simulink library "LIB_TF_G_111"  (Simulink 8.6)
settings: Solver=ode45  StartTime=0.0  StopTime=10.0  RelTol=1e-3
PreLoadFcn:
  | if exist('tl_preloadfcn','file'), tl_preloadfcn(gcs,402); end
PostLoadFcn:
  | if exist('tl_postloadfcn','file'), tl_postloadfcn(gcs,402); end
undefined symbols (not defined in the file or in its folder): ddv
libraries: tllib x1
CloseFcn:
  | if exist('tl_closefcn','file'), tl_closefcn(gcs); end
settings Model: TLRevision=402  Creator=cedric.sauvage  LastModifiedBy=pierre-olivier.pilot

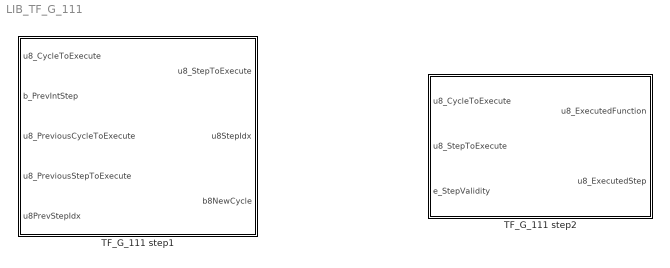
== system LIB_TF_G_111 ==
  TF_G_111 step1 : Subsystem  RequirementInfo={} %GIDa_1baf4a10_21df_4359_ba4d_6c5534378a62  TreatAsAtomicUnit=on
  TF_G_111 step2 : Subsystem  Description=The subsystemDetermineExecutedFunction block is in charge of providing the current executed function output.  RequirementInfo={} %GIDa_d7e9ae14_b57a_42d0_b34c_a685cd16cf1f  TreatAsAtomicUnit=on  RTWFcnName=SelectCycleToExecute
      settings: RTWFcnNameOpts=Use subsystem name

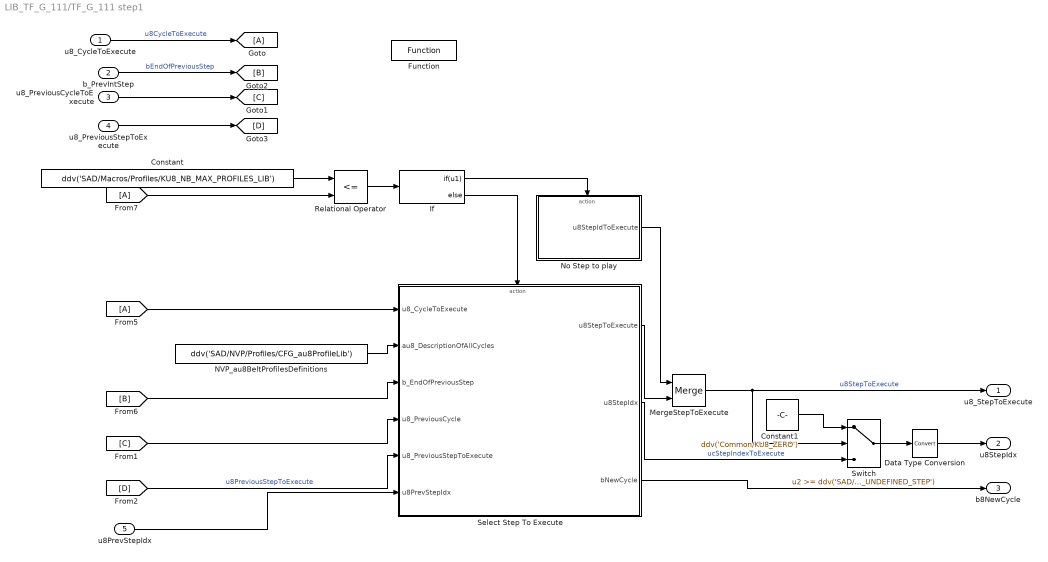
== system LIB_TF_G_111/TF_G_111 step1 ==
  u8_CycleToExecute : Inport  RequirementInfo={} %GIDa_1aab57bb_0326_4cdf_993d_e8a3d032b2dd  PortDimensions=1
  b_PrevIntStep : Inport  RequirementInfo={} %GIDa_baf42ac9_6a3f_411d_a9f1_a6624943f8b6  Port=2  PortDimensions=1
  u8_PreviousCycleToExecute : Inport  RequirementInfo={} %GIDa_c03a94d2_b76b_499f_8873_89e674a9d0bd  Port=3  PortDimensions=1
  u8_PreviousStepToExecute : Inport  RequirementInfo={} %GIDa_366c8ebc_64c9_4731_a983_8ea26311e48e  Port=4  PortDimensions=1
  u8PrevStepIdx : Inport  RequirementInfo={} %GIDa_366c8ebc_64c9_4731_a983_8ea26311e48e  Port=5  PortDimensions=1
  Constant : Constant  RequirementInfo="{}  %GIDa_620c8e9e_71b4_4391_b94d_f5bd98887c44"  Value=ddv('SAD/Macros/Profiles/KU8_NB_MAX_PROFILES_LIB')  OutDataTypeStr=uint8  mask(TL_Constant){data={'output',{'variable','SAD/Macros/Profiles/KU8_NB_MAX_PROFILES_LIB'},'date',738317.72550504631}}
      settings: CopyFcn=if exist('tl_reset_reviewflag','file')==2,tl_reset_reviewflag(gcbh);end  DeleteFcn=if exist('delete_tlblock','file')==2,delete_tlblock(gcbh);end  NameChangeFcn=if exist('rename_tlblock','file')==2,rename_tlblock(gcbh);end  OpenFcn=if exist('tl_open_blockdlg','file')==2,tl_open_blockdlg(gcbh);else,open_system(gcbh,'parameter');end
      mask Help: eval(['if exist(''tl_online_help'',''file'') == 2, tl_online_help(''Topic'',''TL_Constant''),else, web([''jar:file:///'',matlabroot,''/help/toolbox/simulink/help.jar!/slref/' lower(get_param(gcbh,'Blocktype')) '.html''], ''-helpbrowser''),end'])
      mask Display: plot([-0.05, 1.05, NaN, -0.05, 1.05],[.01, .01, NaN, .99, .99])
  Constant1 : Constant  Value=ddv('Common/KU8_ZERO')  mask(TL_Constant){data={'output',{'variable','Common/KU8_ZERO'},'date',738374.40284888889}}
      settings: CopyFcn=if exist('tl_reset_reviewflag') == 2, tl_reset_reviewflag(gcbh); end  DeleteFcn=if exist('delete_tlblock','file')==2,delete_tlblock(gcbh);end  NameChangeFcn=if exist('rename_tlblock','file')==2,rename_tlblock(gcbh);end  OpenFcn=if exist('tl_open_blockdlg','file')==2,tl_open_blockdlg(gcbh);else,open_system(gcbh,'parameter');end
      mask Help: eval(['if exist(''tl_online_help'',''file'') == 2, tl_online_help(''Topic'',''TL_Constant''),else, web([''jar:file:///'',matlabroot,''/help/toolbox/simulink/help.jar!/slref/' lower(get_param(gcbh,'Blocktype')) '.html''], ''-helpbrowser''),end'])
      mask Display: plot([-0.1, 1.05, NaN, -0.1, 1.05],[.01, .01, NaN, .99, .99]);
  Data Type Conversion : DataTypeConversion
  Function : tllib/Function  RequirementInfo={'other' '..\..\..\..\Documents and Settings\cedric.sauvage\Desktop\BFE_Design.doc' '@Simulink_requirement_item_11' 'true' 'DSG_BFE_00022' '' } %GIDa_e008078b_e0b8_4be4_b617_b81ec49ed686  data={'stepfunctionname','M_SelectStepId','stepfunctionclass','STATIC_FCN','restartfunctionname','RESTART_$S','initfunctionname','INIT_$S','termfunctionname','TERM_$S','subsystemid','b','codecomment',['[COVERS: DSG_BFE_00022]'],'date',738317.71884769679}  displayString=FUNCTION
  If : If  RequirementInfo="{}  %GIDa_294fbd4d_f0d9_4546_9a6f_38fd5f5ce9cd"  IfExpression=u1
  MergeStepToExecute : Merge  RequirementInfo={} %GIDa_00bbe0bd_4739_4f59_a29d_488204ffbd9c  InitialOutput=255  mask(TL_Merge){data={'comment',{'text',['Variable to store the Step Id that will be executed.' char(10) 'Range : [0 ; 7 ] U {255}']},'logdata',{'loggingmode',1},'output',{'name','u8StepToExecute','type','UInt8','inheritscaling',0},'autoscaling',{'mode',2},'date',738342.71431006945}}
      settings: CopyFcn=if exist('tl_reset_reviewflag','file')==2,tl_reset_reviewflag(gcbh);end  DeleteFcn=if exist('delete_tlblock','file')==2,delete_tlblock(gcbh);end  NameChangeFcn=if exist('rename_tlblock','file')==2,rename_tlblock(gcbh);end  OpenFcn=if exist('tl_open_blockdlg','file')==2,tl_open_blockdlg(gcbh);else,open_system(gcbh,'parameter');end
      mask Help: eval(['if exist(''tl_online_help'',''file'') == 2, tl_online_help(''Topic'',''TL_Merge''),else, web([''jar:file:///'',matlabroot,''/help/toolbox/simulink/help.jar!/slref/' lower(get_param(gcbh,'Blocktype')) '.html''], ''-helpbrowser''),end'])
      mask Display: plot([-0.05, 1.05, NaN, -0.05, 1.05],[.01, .01, NaN, .99, .99])
  NVP_au8BeltProfilesDefinitions : Constant  RequirementInfo={} %GIDa_2310f87e_6155_40ae_92aa_a4e85bb40bf8  Value=ddv('SAD/NVP/Profiles/CFG_au8ProfileLib')  OutDataTypeStr=uint8  SampleTime=-1  mask(TL_Constant){data={'output',{'variable','SAD/NVP/Profiles/CFG_au8ProfileLib'},'autoscaling',{'mode',2,'scalingvalid',1},'date',738317.72849901626}}
      settings: CopyFcn=if exist('tl_reset_reviewflag','file')==2,tl_reset_reviewflag(gcbh);end  DeleteFcn=if exist('delete_tlblock','file')==2,delete_tlblock(gcbh);end  NameChangeFcn=if exist('rename_tlblock','file')==2,rename_tlblock(gcbh);end  OpenFcn=if exist('tl_open_blockdlg','file')==2,tl_open_blockdlg(gcbh);else,open_system(gcbh,'parameter');end
      mask Help: eval(['if exist(''tl_online_help'',''file'') == 2, tl_online_help(''Topic'',''TL_Constant''),else, web([''jar:file:///'',matlabroot,''/help/toolbox/simulink/help.jar!/slref/' lower(get_param(gcbh,'Blocktype')) '.html''], ''-helpbrowser''),end'])
      mask Display: plot([-0.05, 1.05, NaN, -0.05, 1.05],[.01, .01, NaN, .99, .99])
  No Step to play : Subsystem  RequirementInfo={} %GIDa_d91b2e4f_18cc_4d88_b22a_15159c806b5d  TreatAsAtomicUnit=on
  Relational Operator : RelationalOperator  RequirementInfo="{}  %GIDa_efbacf4c_d6af_4eb6_a19c_9e619873ad52"  Operator=<=  OutDataTypeStr=boolean  mask(TL_RelationalOperator){data={'output',{'name','bIsValidCycle'},'date',735951.66832363431}}
      settings: DeleteFcn=if exist('delete_tlblock','file')==2,delete_tlblock(gcbh);end  NameChangeFcn=if exist('rename_tlblock','file')==2,rename_tlblock(gcbh);end  OpenFcn=if exist('tl_open_blockdlg','file')==2,tl_open_blockdlg(gcbh);else,open_system(gcbh,'parameter');end
      mask Help: eval(['if exist(''tl_online_help'',''file'') == 2, tl_online_help(''Topic'',''TL_RelationalOperator''),else, web([''jar:file:///'',matlabroot,''/help/toolbox/simulink/help.jar!/slref/' lower(get_param(gcbh,'Blocktype')) '.html''], ''-helpbrowser''),end'])
      mask Display: plot([-0.05, 1.05, NaN, -0.05, 1.05],[.01, .01, NaN, .99, .99])
  Select Step To Execute : Subsystem  RequirementInfo={} %GIDa_31ce642c_6a48_44ac_acee_58c46d748f2b  TreatAsAtomicUnit=on  RTWFcnName=SelectStepToExecute
      settings: RTWFcnNameOpts=Use subsystem name
  Switch : Switch  Threshold=ddv('SAD/Macros/Steps/KUC_UNDEFINED_STEP')  mask(TL_Switch){data={'output',{'type','UInt8'},'threshold',{'variable','SAD/Macros/Steps/KUC_UNDEFINED_STEP'},'date',738374.39737903932}}
      settings: CopyFcn=if exist('tl_reset_reviewflag') == 2, tl_reset_reviewflag(gcbh); end  DeleteFcn=if exist('delete_tlblock','file')==2,delete_tlblock(gcbh);end  NameChangeFcn=if exist('rename_tlblock','file')==2,rename_tlblock(gcbh);end  OpenFcn=if exist('tl_open_blockdlg','file')==2,tl_open_blockdlg(gcbh);else,open_system(gcbh,'parameter');end
      mask Help: eval(['if exist(''tl_online_help'',''file'') == 2, tl_online_help(''Topic'',''TL_Switch''),else, web([''jar:file:///'',matlabroot,''/help/toolbox/simulink/help.jar!/slref/' lower(get_param(gcbh,'Blocktype')) '.html''], ''-helpbrowser''),end'])
      mask Display: plot([-0.1, 1.05, NaN, -0.1, 1.05],[.01, .01, NaN, .99, .99]);
  u8_StepToExecute : Outport  RequirementInfo={} %GIDa_adc63fab_a360_486b_a74e_418a5d4fa8d3  PortDimensions=1
  u8StepIdx : Outport  RequirementInfo={} %GIDa_adc63fab_a360_486b_a74e_418a5d4fa8d3  Port=2  PortDimensions=1
  b8NewCycle : Outport  RequirementInfo={} %GIDa_adc63fab_a360_486b_a74e_418a5d4fa8d3  Port=3  PortDimensions=1
  wires:
  MergeStepToExecute/1 -> Switch/2, u8_StepToExecute/1  "u8StepToExecute"
  Select Step To Execute/1(u8StepToExecute) -> MergeStepToExecute/2
  NVP_au8BeltProfilesDefinitions/1 -> Select Step To Execute/2(au8_DescriptionOfAllCycles)
  [D] -> Select Step To Execute/5(u8_PreviousStepToExecute)  "u8PreviousStepToExecute"
  [C] -> Select Step To Execute/4(u8_PreviousCycle)
  b_PrevIntStep/1 -> [B]  "bEndOfPreviousStep"
  [A] -> Select Step To Execute/1(u8_CycleToExecute)
  [B] -> Select Step To Execute/3(b_EndOfPreviousStep)
  If/1 -> No Step to play/Action
  Constant/1 -> Relational Operator/1
  [A] -> Relational Operator/2
  Relational Operator/1 -> If/1
  If/2 -> Select Step To Execute/Action
  No Step to play/1(u8StepIdToExecute) -> MergeStepToExecute/1
  u8_PreviousCycleToExecute/1 -> [C]
  u8_PreviousStepToExecute/1 -> [D]
  u8PrevStepIdx/1 -> Select Step To Execute/6(u8PrevStepIdx)
  Switch/1 -> Data Type Conversion/1
  Select Step To Execute/2(u8StepIdx) -> Switch/3  "ucStepIndexToExecute"
  Data Type Conversion/1 -> u8StepIdx/1
  Constant1/1 -> Switch/1
  Select Step To Execute/3(bNewCycle) -> b8NewCycle/1
  u8_CycleToExecute/1 -> [A]  "u8CycleToExecute"

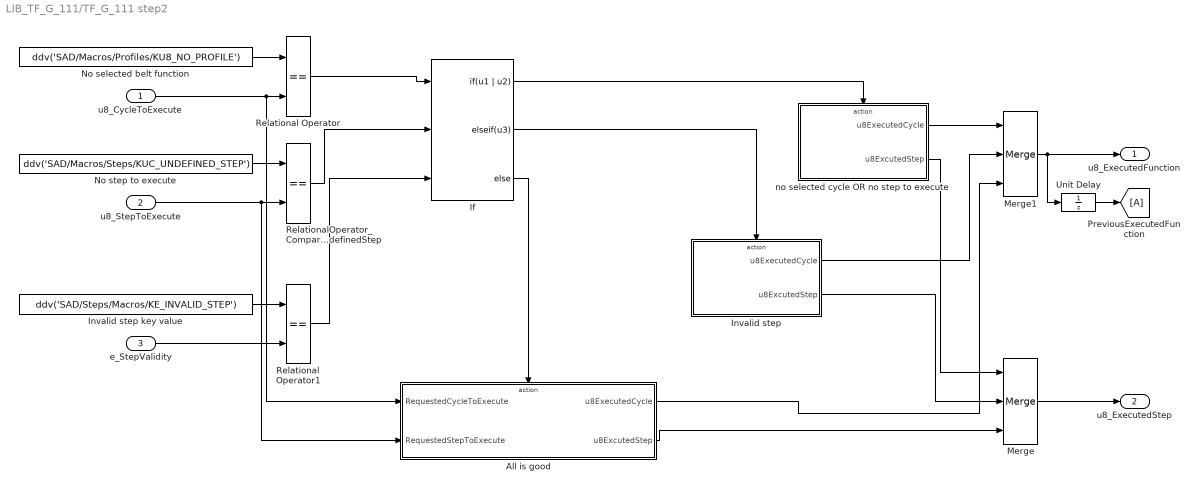
== system LIB_TF_G_111/TF_G_111 step2 ==
  u8_CycleToExecute : Inport  RequirementInfo={} %GIDa_8fea8efb_b987_405d_b9e8_745dfc9acb95
  u8_StepToExecute : Inport  RequirementInfo={} %GIDa_61957716_bf53_4143_936d_c46b278fe403  Port=2  OutDataTypeStr=uint8
  e_StepValidity : Inport  RequirementInfo={} %GIDa_5e092c6c_cd76_45bb_8082_3f7ed93fce89  Port=3
  All is good : Subsystem  TreatAsAtomicUnit=on
  If : If  NumInputs=3  IfExpression=u1 | u2  ElseIfExpressions=u3
  Invalid step : Subsystem  TreatAsAtomicUnit=on
  Invalid step key value : Constant  RequirementInfo={} %GIDa_416a43f8_dea2_4baf_bffb_a83f416ddf80  Value=ddv('SAD/Steps/Macros/KE_INVALID_STEP')  OutDataTypeStr=Inherit: Inherit via back propagation  mask(TL_Constant){data={'output',{'variable','SAD/Steps/Macros/KE_INVALID_STEP'},'date',738321.62849513884}}
      settings: CopyFcn=if exist('tl_reset_reviewflag','file')==2,tl_reset_reviewflag(gcbh);end  DeleteFcn=if exist('delete_tlblock','file')==2,delete_tlblock(gcbh);end  NameChangeFcn=if exist('rename_tlblock','file')==2,rename_tlblock(gcbh);end  OpenFcn=if exist('tl_open_blockdlg','file')==2,tl_open_blockdlg(gcbh);else,open_system(gcbh,'parameter');end
      mask Help: eval(['if exist(''tl_online_help'',''file'') == 2, tl_online_help(''Topic'',''TL_Constant''),else, web([''jar:file:///'',matlabroot,''/help/toolbox/simulink/help.jar!/slref/' lower(get_param(gcbh,'Blocktype')) '.html''], ''-helpbrowser''),end'])
      mask Display: plot([-0.05, 1.05, NaN, -0.05, 1.05],[.01, .01, NaN, .99, .99])
  Merge : Merge  Inputs=3  InitialOutput=255  mask(TL_Merge){data={'output',{'name','u8ExecutedStep'},'date',738321.62694715278}}
      settings: CopyFcn=if exist('tl_reset_reviewflag','file')==2,tl_reset_reviewflag(gcbh);end  DeleteFcn=if exist('delete_tlblock','file')==2,delete_tlblock(gcbh);end  NameChangeFcn=if exist('rename_tlblock','file')==2,rename_tlblock(gcbh);end  OpenFcn=if exist('tl_open_blockdlg','file')==2,tl_open_blockdlg(gcbh);else,open_system(gcbh,'parameter');end
      mask Help: eval(['if exist(''tl_online_help'',''file'') == 2, tl_online_help(''Topic'',''TL_Merge''),else, web([''jar:file:///'',matlabroot,''/help/toolbox/simulink/help.jar!/slref/' lower(get_param(gcbh,'Blocktype')) '.html''], ''-helpbrowser''),end'])
      mask Display: plot([-0.05, 1.05, NaN, -0.05, 1.05],[.01, .01, NaN, .99, .99])
  Merge1 : Merge  Inputs=3  InitialOutput=255  mask(TL_Merge){data={'output',{'name','u8ExecutedCycle'},'date',738321.62687034719}}
      settings: CopyFcn=if exist('tl_reset_reviewflag','file')==2,tl_reset_reviewflag(gcbh);end  DeleteFcn=if exist('delete_tlblock','file')==2,delete_tlblock(gcbh);end  NameChangeFcn=if exist('rename_tlblock','file')==2,rename_tlblock(gcbh);end  OpenFcn=if exist('tl_open_blockdlg','file')==2,tl_open_blockdlg(gcbh);else,open_system(gcbh,'parameter');end
      mask Help: eval(['if exist(''tl_online_help'',''file'') == 2, tl_online_help(''Topic'',''TL_Merge''),else, web([''jar:file:///'',matlabroot,''/help/toolbox/simulink/help.jar!/slref/' lower(get_param(gcbh,'Blocktype')) '.html''], ''-helpbrowser''),end'])
      mask Display: plot([-0.05, 1.05, NaN, -0.05, 1.05],[.01, .01, NaN, .99, .99])
  No selected belt function : Constant  RequirementInfo={} %GIDa_4bc26cfd_c29d_4ec8_a88f_554466473695  Value=ddv('SAD/Macros/Profiles/KU8_NO_PROFILE')  OutDataTypeStr=uint8  mask(TL_Constant){data={'output',{'variable','SAD/Macros/Profiles/KU8_NO_PROFILE'},'date',738321.62805532408}}
      settings: CopyFcn=if exist('tl_reset_reviewflag','file')==2,tl_reset_reviewflag(gcbh);end  DeleteFcn=if exist('delete_tlblock','file')==2,delete_tlblock(gcbh);end  NameChangeFcn=if exist('rename_tlblock','file')==2,rename_tlblock(gcbh);end  OpenFcn=if exist('tl_open_blockdlg','file')==2,tl_open_blockdlg(gcbh);else,open_system(gcbh,'parameter');end
      mask Help: eval(['if exist(''tl_online_help'',''file'') == 2, tl_online_help(''Topic'',''TL_Constant''),else, web([''jar:file:///'',matlabroot,''/help/toolbox/simulink/help.jar!/slref/' lower(get_param(gcbh,'Blocktype')) '.html''], ''-helpbrowser''),end'])
      mask Display: plot([-0.05, 1.05, NaN, -0.05, 1.05],[.01, .01, NaN, .99, .99])
  No step to execute : Constant  RequirementInfo={} %GIDa_8bc1bd8d_9fc4_41ed_9f7f_2899e2e1c57d  Value=ddv('SAD/Macros/Steps/KUC_UNDEFINED_STEP')  OutDataTypeStr=Inherit: Inherit via back propagation  mask(TL_Constant){data={'output',{'variable','SAD/Macros/Steps/KUC_UNDEFINED_STEP'},'date',738321.62822025467}}
      settings: CopyFcn=if exist('tl_reset_reviewflag','file')==2,tl_reset_reviewflag(gcbh);end  DeleteFcn=if exist('delete_tlblock','file')==2,delete_tlblock(gcbh);end  NameChangeFcn=if exist('rename_tlblock','file')==2,rename_tlblock(gcbh);end  OpenFcn=if exist('tl_open_blockdlg','file')==2,tl_open_blockdlg(gcbh);else,open_system(gcbh,'parameter');end
      mask Help: eval(['if exist(''tl_online_help'',''file'') == 2, tl_online_help(''Topic'',''TL_Constant''),else, web([''jar:file:///'',matlabroot,''/help/toolbox/simulink/help.jar!/slref/' lower(get_param(gcbh,'Blocktype')) '.html''], ''-helpbrowser''),end'])
      mask Display: plot([-0.05, 1.05, NaN, -0.05, 1.05],[.01, .01, NaN, .99, .99])
  Relational Operator : RelationalOperator  Operator===  OutDataTypeStr=boolean  mask(TL_RelationalOperator){data={'date',735951.66831112269}}
      settings: DeleteFcn=if exist('delete_tlblock','file')==2,delete_tlblock(gcbh);end  NameChangeFcn=if exist('rename_tlblock','file')==2,rename_tlblock(gcbh);end  OpenFcn=if exist('tl_open_blockdlg','file')==2,tl_open_blockdlg(gcbh);else,open_system(gcbh,'parameter');end
      mask Help: eval(['if exist(''tl_online_help'',''file'') == 2, tl_online_help(''Topic'',''TL_RelationalOperator''),else, web([''jar:file:///'',matlabroot,''/help/toolbox/simulink/help.jar!/slref/' lower(get_param(gcbh,'Blocktype')) '.html''], ''-helpbrowser''),end'])
      mask Display: plot([-0.05, 1.05, NaN, -0.05, 1.05],[.01, .01, NaN, .99, .99])
  Relational Operator1 : RelationalOperator  Operator===  OutDataTypeStr=boolean  mask(TL_RelationalOperator){data={'date',735951.66831087961}}
      settings: DeleteFcn=if exist('delete_tlblock','file')==2,delete_tlblock(gcbh);end  NameChangeFcn=if exist('rename_tlblock','file')==2,rename_tlblock(gcbh);end  OpenFcn=if exist('tl_open_blockdlg','file')==2,tl_open_blockdlg(gcbh);else,open_system(gcbh,'parameter');end
      mask Help: eval(['if exist(''tl_online_help'',''file'') == 2, tl_online_help(''Topic'',''TL_RelationalOperator''),else, web([''jar:file:///'',matlabroot,''/help/toolbox/simulink/help.jar!/slref/' lower(get_param(gcbh,'Blocktype')) '.html''], ''-helpbrowser''),end'])
      mask Display: plot([-0.05, 1.05, NaN, -0.05, 1.05],[.01, .01, NaN, .99, .99])
  RelationalOperator_CompareToUndefinedStep : RelationalOperator  RequirementInfo={} %GIDa_4071e895_5093_4781_8864_58a78a6d4067  Operator===  OutDataTypeStr=boolean  mask(TL_RelationalOperator){data={'date',735951.66831063654}}
      settings: DeleteFcn=if exist('delete_tlblock','file')==2,delete_tlblock(gcbh);end  NameChangeFcn=if exist('rename_tlblock','file')==2,rename_tlblock(gcbh);end  OpenFcn=if exist('tl_open_blockdlg','file')==2,tl_open_blockdlg(gcbh);else,open_system(gcbh,'parameter');end
      mask Help: eval(['if exist(''tl_online_help'',''file'') == 2, tl_online_help(''Topic'',''TL_RelationalOperator''),else, web([''jar:file:///'',matlabroot,''/help/toolbox/simulink/help.jar!/slref/' lower(get_param(gcbh,'Blocktype')) '.html''], ''-helpbrowser''),end'])
      mask Display: plot([-0.05, 1.05, NaN, -0.05, 1.05],[.01, .01, NaN, .99, .99])
  Unit Delay : UnitDelay  InitialCondition=255  SampleTime=-1  mask(TL_UnitDelay){data={'output',{'type','UInt8'},'state',{'name','u8PreviousExecutedFunction','type','UInt8'},'date',735951.66831032408}}
      settings: CopyFcn=if exist('tl_reset_reviewflag','file')==2,tl_reset_reviewflag(gcbh);end  DeleteFcn=if exist('delete_tlblock','file')==2,delete_tlblock(gcbh);end  NameChangeFcn=if exist('rename_tlblock','file')==2,rename_tlblock(gcbh);end  OpenFcn=if exist('tl_open_blockdlg','file')==2,tl_open_blockdlg(gcbh);else,open_system(gcbh,'parameter');end
      mask Help: eval(['if exist(''tl_online_help'',''file'') == 2, tl_online_help(''Topic'',''TL_UnitDelay''),else, web([''jar:file:///'',matlabroot,''/help/toolbox/simulink/help.jar!/slref/' lower(get_param(gcbh,'Blocktype')) '.html''], ''-helpbrowser''),end'])
      mask Display: plot([-0.05, 1.05, NaN, -0.05, 1.05],[.01, .01, NaN, .99, .99])
  no selected cycle OR no step to execute : Subsystem  TreatAsAtomicUnit=on
  u8_ExecutedFunction : Outport  RequirementInfo={} %GIDa_8713064f_f4a9_42db_8bb1_59bc8ff89bda
  u8_ExecutedStep : Outport  RequirementInfo={} %GIDa_27e8687a_de30_4ff7_b10f_aecac094b4c1  Port=2
  wires:
  No selected belt function/1 -> Relational Operator/1
  u8_CycleToExecute/1 -> Relational Operator/2, All is good/1(RequestedCycleToExecute)
  No step to execute/1 -> RelationalOperator_CompareToUndefinedStep/1
  u8_StepToExecute/1 -> RelationalOperator_CompareToUndefinedStep/2, All is good/2(RequestedStepToExecute)
  If/1 -> no selected cycle OR no step to execute/Action
  Relational Operator/1 -> If/1
  RelationalOperator_CompareToUndefinedStep/1 -> If/2
  e_StepValidity/1 -> Relational Operator1/2
  Relational Operator1/1 -> If/3
  Invalid step key value/1 -> Relational Operator1/1
  If/2 -> Invalid step/Action
  If/3 -> All is good/Action
  Merge1/1 -> u8_ExecutedFunction/1, Unit Delay/1
  Merge/1 -> u8_ExecutedStep/1
  no selected cycle OR no step to execute/1(u8ExecutedCycle) -> Merge1/1
  Invalid step/1(u8ExecutedCycle) -> Merge1/2
  All is good/1(u8ExecutedCycle) -> Merge1/3
  All is good/2(u8ExcutedStep) -> Merge/3
  Invalid step/2(u8ExcutedStep) -> Merge/2
  no selected cycle OR no step to execute/2(u8ExcutedStep) -> Merge/1
  Unit Delay/1 -> [A]

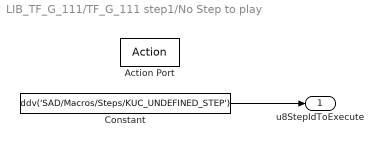
== system LIB_TF_G_111/TF_G_111 step1/No Step to play ==
  Action Port : ActionPort  RequirementInfo="{}  %GIDa_9b0f36a1_581d_4938_a95d_cea0f15c05a5"
  Constant : Constant  RequirementInfo="{}  %GIDa_afeedc86_4d10_4281_9703_4ed2f747546e"  Value=ddv('SAD/Macros/Steps/KUC_UNDEFINED_STEP')  OutDataTypeStr=uint8  mask(TL_Constant){data={'output',{'variable','SAD/Macros/Steps/KUC_UNDEFINED_STEP'},'date',738321.62035557872}}
      settings: CopyFcn=if exist('tl_reset_reviewflag','file')==2,tl_reset_reviewflag(gcbh);end  DeleteFcn=if exist('delete_tlblock','file')==2,delete_tlblock(gcbh);end  NameChangeFcn=if exist('rename_tlblock','file')==2,rename_tlblock(gcbh);end  OpenFcn=if exist('tl_open_blockdlg','file')==2,tl_open_blockdlg(gcbh);else,open_system(gcbh,'parameter');end
      mask Help: eval(['if exist(''tl_online_help'',''file'') == 2, tl_online_help(''Topic'',''TL_Constant''),else, web([''jar:file:///'',matlabroot,''/help/toolbox/simulink/help.jar!/slref/' lower(get_param(gcbh,'Blocktype')) '.html''], ''-helpbrowser''),end'])
      mask Display: plot([-0.05, 1.05, NaN, -0.05, 1.05],[.01, .01, NaN, .99, .99])
  u8StepIdToExecute : Outport  RequirementInfo={} %GIDa_e4a2b18c_09f1_4793_aba0_5f1c3953a216  InitialOutput=255
  wires:
  Constant/1 -> u8StepIdToExecute/1

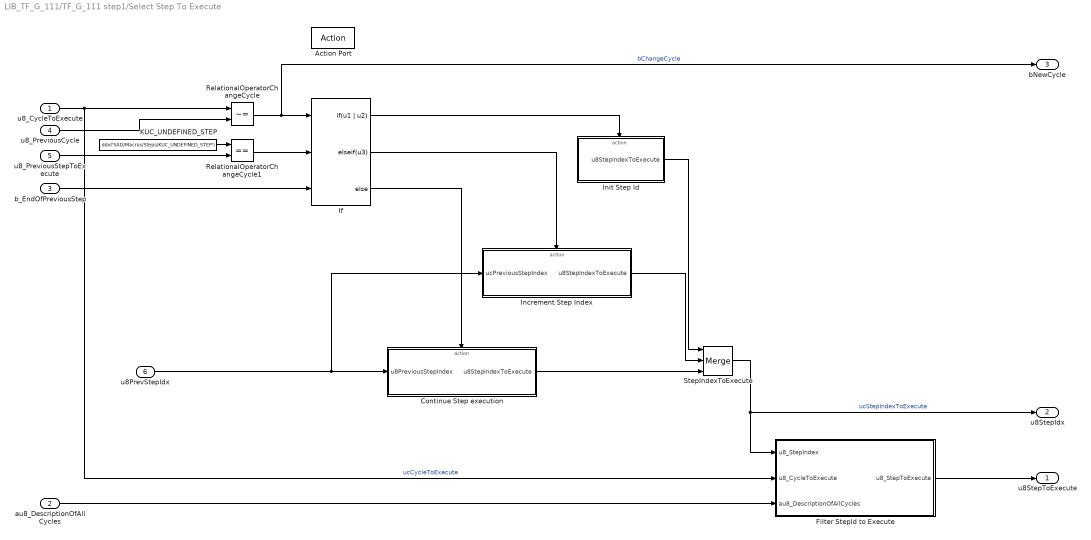
== system LIB_TF_G_111/TF_G_111 step1/Select Step To Execute ==
  u8_CycleToExecute : Inport  RequirementInfo={} %GIDa_8d4e5bab_b80e_4e01_81ce_b6e790b131fb
  au8_DescriptionOfAllCycles : Inport  RequirementInfo={} %GIDa_c06da474_c08f_46d9_92bb_9088ec013155  Port=2  OutDataTypeStr=uint8
  b_EndOfPreviousStep : Inport  RequirementInfo={} %GIDa_2c1722e4_980a_48a1_8990_301358730051  Port=3
  u8_PreviousCycle : Inport  RequirementInfo={} %GIDa_7ceb08ad_35fc_4b74_8f3b_a28497a2e219  Port=4
  u8_PreviousStepToExecute : Inport  RequirementInfo={} %GIDa_3793ab51_f047_4f43_8cee_9c5d044f6ee6  Port=5
  u8PrevStepIdx : Inport  RequirementInfo={} %GIDa_c06da474_c08f_46d9_92bb_9088ec013155  Port=6
  Action Port : ActionPort  RequirementInfo="{}  %GIDa_ec02541f_ac93_4bf3_836c_122371ae3eb9"
  Continue Step execution : Subsystem  RequirementInfo={} %GIDa_567d5d98_645d_41b3_b901_4f423276d610  TreatAsAtomicUnit=on
      settings: RTWFcnNameOpts=Use subsystem name
  Filter StepId to Execute : Subsystem  RequirementInfo="{}  %GIDa_085e2bbf_61cb_45fc_84b4_da4c9f215240"  TreatAsAtomicUnit=on
  If : If  RequirementInfo="{}  %GIDa_fe303313_68dd_49c9_a488_ab8c67144df8"  NumInputs=3  IfExpression=u1 | u2  ElseIfExpressions=u3
  Increment Step Index : Subsystem  RequirementInfo={} %GIDa_2230e77a_bf9c_4d74_97b3_452ba0c63b0a  TreatAsAtomicUnit=on
      settings: RTWFcnNameOpts=Use subsystem name
  Init Step Id : Subsystem  RequirementInfo={} %GIDa_4cdf07f5_0d4f_4f30_b6c8_d016748c9874  TreatAsAtomicUnit=on
      settings: RTWFcnNameOpts=Use subsystem name
  KUC_UNDEFINED_STEP : Constant  RequirementInfo={} %GIDa_15357e27_e5c7_4390_bd4f_b839d31ef5c6  Value=ddv('SAD/Macros/Steps/KUC_UNDEFINED_STEP')  OutDataTypeStr=uint8  mask(TL_Constant){data={'output',{'variable','SAD/Macros/Steps/KUC_UNDEFINED_STEP'},'date',738321.62077575235}}
      settings: CopyFcn=if exist('tl_reset_reviewflag','file')==2,tl_reset_reviewflag(gcbh);end  DeleteFcn=if exist('delete_tlblock','file')==2,delete_tlblock(gcbh);end  NameChangeFcn=if exist('rename_tlblock','file')==2,rename_tlblock(gcbh);end  OpenFcn=if exist('tl_open_blockdlg','file')==2,tl_open_blockdlg(gcbh);else,open_system(gcbh,'parameter');end
      mask Help: eval(['if exist(''tl_online_help'',''file'') == 2, tl_online_help(''Topic'',''TL_Constant''),else, web([''jar:file:///'',matlabroot,''/help/toolbox/simulink/help.jar!/slref/' lower(get_param(gcbh,'Blocktype')) '.html''], ''-helpbrowser''),end'])
      mask Display: plot([-0.05, 1.05, NaN, -0.05, 1.05],[.01, .01, NaN, .99, .99])
  RelationalOperatorChangeCycle : RelationalOperator  RequirementInfo={} %GIDa_0c82807a_81d1_42ec_adac_a2f1c288664a  Operator=~=  OutDataTypeStr=boolean  ZeroCross=off  mask(TL_RelationalOperator){data={'output',{'name','bHasCycleChanged'},'date',735951.66831762728}}
      settings: DeleteFcn=if exist('delete_tlblock','file')==2,delete_tlblock(gcbh);end  NameChangeFcn=if exist('rename_tlblock','file')==2,rename_tlblock(gcbh);end  OpenFcn=if exist('tl_open_blockdlg','file')==2,tl_open_blockdlg(gcbh);else,open_system(gcbh,'parameter');end
      mask Help: eval(['if exist(''tl_online_help'',''file'') == 2, tl_online_help(''Topic'',''TL_RelationalOperator''),else, web([''jar:file:///'',matlabroot,''/help/toolbox/simulink/help.jar!/slref/' lower(get_param(gcbh,'Blocktype')) '.html''], ''-helpbrowser''),end'])
      mask Display: plot([-0.05, 1.05, NaN, -0.05, 1.05],[.01, .01, NaN, .99, .99])
  RelationalOperatorChangeCycle1 : RelationalOperator  RequirementInfo={} %GIDa_c96d9746_f8c6_4abd_a58c_f9e69e7c3389  Operator===  OutDataTypeStr=boolean  ZeroCross=off  mask(TL_RelationalOperator){data={'date',735951.66831736115}}
      settings: DeleteFcn=if exist('delete_tlblock','file')==2,delete_tlblock(gcbh);end  NameChangeFcn=if exist('rename_tlblock','file')==2,rename_tlblock(gcbh);end  OpenFcn=if exist('tl_open_blockdlg','file')==2,tl_open_blockdlg(gcbh);else,open_system(gcbh,'parameter');end
      mask Help: eval(['if exist(''tl_online_help'',''file'') == 2, tl_online_help(''Topic'',''TL_RelationalOperator''),else, web([''jar:file:///'',matlabroot,''/help/toolbox/simulink/help.jar!/slref/' lower(get_param(gcbh,'Blocktype')) '.html''], ''-helpbrowser''),end'])
      mask Display: plot([-0.05, 1.05, NaN, -0.05, 1.05],[.01, .01, NaN, .99, .99])
  StepIndexToExecute : Merge  RequirementInfo={} %GIDa_1b7985cc_8fad_4670_b396_0d4aca6974d8  Inputs=3  InitialOutput=255  mask(TL_Merge){data={'output',{'name','u8UnfilteredStepId'},'date',735951.66831707174}}
      settings: CopyFcn=if exist('tl_reset_reviewflag','file')==2,tl_reset_reviewflag(gcbh);end  DeleteFcn=if exist('delete_tlblock','file')==2,delete_tlblock(gcbh);end  NameChangeFcn=if exist('rename_tlblock','file')==2,rename_tlblock(gcbh);end  OpenFcn=if exist('tl_open_blockdlg','file')==2,tl_open_blockdlg(gcbh);else,open_system(gcbh,'parameter');end
      mask Help: eval(['if exist(''tl_online_help'',''file'') == 2, tl_online_help(''Topic'',''TL_Merge''),else, web([''jar:file:///'',matlabroot,''/help/toolbox/simulink/help.jar!/slref/' lower(get_param(gcbh,'Blocktype')) '.html''], ''-helpbrowser''),end'])
      mask Display: plot([-0.05, 1.05, NaN, -0.05, 1.05],[.01, .01, NaN, .99, .99])
  u8StepToExecute : Outport  RequirementInfo={} %GIDa_433c26c1_7119_4ede_b400_eae74db2e302  InitialOutput=255
  u8StepIdx : Outport  RequirementInfo={} %GIDa_433c26c1_7119_4ede_b400_eae74db2e302  Port=2  InitialOutput=255
  bNewCycle : Outport  RequirementInfo={} %GIDa_433c26c1_7119_4ede_b400_eae74db2e302  Port=3  InitialOutput=0
  wires:
  b_EndOfPreviousStep/1 -> If/3
  StepIndexToExecute/1 -> Filter StepId to Execute/1(u8_StepIndex), u8StepIdx/1  "ucStepIndexToExecute"
  Increment Step Index/1(u8StepIndexToExecute) -> StepIndexToExecute/2
  u8_CycleToExecute/1 -> RelationalOperatorChangeCycle/1, Filter StepId to Execute/2(u8_CycleToExecute)  "ucCycleToExecute"
  Init Step Id/1(u8StepIndexToExecute) -> StepIndexToExecute/1
  u8_PreviousCycle/1 -> RelationalOperatorChangeCycle/2
  u8_PreviousStepToExecute/1 -> RelationalOperatorChangeCycle1/2
  RelationalOperatorChangeCycle/1 -> bNewCycle/1, If/1  "bChangeCycle"
  If/1 -> Init Step Id/Action
  If/2 -> Increment Step Index/Action
  If/3 -> Continue Step execution/Action
  KUC_UNDEFINED_STEP/1 -> RelationalOperatorChangeCycle1/1
  RelationalOperatorChangeCycle1/1 -> If/2
  Continue Step execution/1(u8StepIndexToExecute) -> StepIndexToExecute/3
  au8_DescriptionOfAllCycles/1 -> Filter StepId to Execute/3(au8_DescriptionOfAllCycles)
  u8PrevStepIdx/1 -> Increment Step Index/1(ucPreviousStepIndex), Continue Step execution/1(u8PreviousStepIndex)
  Filter StepId to Execute/1(u8_StepToExecute) -> u8StepToExecute/1

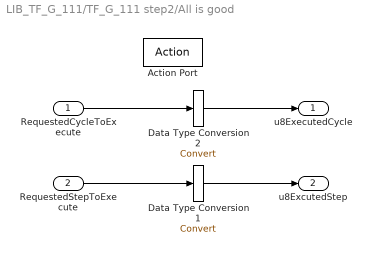
== system LIB_TF_G_111/TF_G_111 step2/All is good ==
  RequestedCycleToExecute : Inport  RequirementInfo={} %GIDa_c6656af6_5dc6_4240_9dfe_354d08ac5268
  RequestedStepToExecute : Inport  RequirementInfo={} %GIDa_947e64c1_bf3b_4bd6_a910_13dfd1c197d6  Port=2  OutDataTypeStr=uint8
  Action Port : ActionPort  ActionType=else
  Data Type Conversion1 : DataTypeConversion
  Data Type Conversion2 : DataTypeConversion
  u8ExecutedCycle : Outport
  u8ExcutedStep : Outport  Port=2
  wires:
  RequestedCycleToExecute/1 -> Data Type Conversion2/1
  RequestedStepToExecute/1 -> Data Type Conversion1/1
  Data Type Conversion2/1 -> u8ExecutedCycle/1
  Data Type Conversion1/1 -> u8ExcutedStep/1

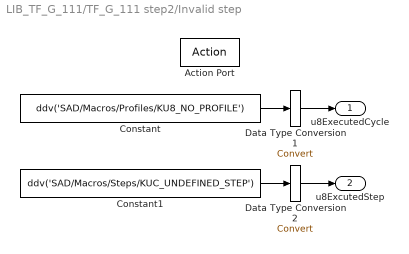
== system LIB_TF_G_111/TF_G_111 step2/Invalid step ==
  Action Port : ActionPort  ActionType=elseif
  Constant : Constant  Value=ddv('SAD/Macros/Profiles/KU8_NO_PROFILE')  mask(TL_Constant){data={'output',{'variable','SAD/Macros/Profiles/KU8_NO_PROFILE'},'date',738321.62969498837}}
      settings: CopyFcn=if exist('tl_reset_reviewflag','file')==2,tl_reset_reviewflag(gcbh);end  DeleteFcn=if exist('delete_tlblock','file')==2,delete_tlblock(gcbh);end  NameChangeFcn=if exist('rename_tlblock','file')==2,rename_tlblock(gcbh);end  OpenFcn=if exist('tl_open_blockdlg','file')==2,tl_open_blockdlg(gcbh);else,open_system(gcbh,'parameter');end
      mask Help: eval(['if exist(''tl_online_help'',''file'') == 2, tl_online_help(''Topic'',''TL_Constant''),else, web([''jar:file:///'',matlabroot,''/help/toolbox/simulink/help.jar!/slref/' lower(get_param(gcbh,'Blocktype')) '.html''], ''-helpbrowser''),end'])
      mask Display: plot([-0.05, 1.05, NaN, -0.05, 1.05],[.01, .01, NaN, .99, .99])
  Constant1 : Constant  Value=ddv('SAD/Macros/Steps/KUC_UNDEFINED_STEP')  mask(TL_Constant){data={'output',{'variable','SAD/Macros/Steps/KUC_UNDEFINED_STEP'},'date',738321.62986325228}}
      settings: CopyFcn=if exist('tl_reset_reviewflag','file')==2,tl_reset_reviewflag(gcbh);end  DeleteFcn=if exist('delete_tlblock','file')==2,delete_tlblock(gcbh);end  NameChangeFcn=if exist('rename_tlblock','file')==2,rename_tlblock(gcbh);end  OpenFcn=if exist('tl_open_blockdlg','file')==2,tl_open_blockdlg(gcbh);else,open_system(gcbh,'parameter');end
      mask Help: eval(['if exist(''tl_online_help'',''file'') == 2, tl_online_help(''Topic'',''TL_Constant''),else, web([''jar:file:///'',matlabroot,''/help/toolbox/simulink/help.jar!/slref/' lower(get_param(gcbh,'Blocktype')) '.html''], ''-helpbrowser''),end'])
      mask Display: plot([-0.05, 1.05, NaN, -0.05, 1.05],[.01, .01, NaN, .99, .99])
  Data Type Conversion1 : DataTypeConversion
  Data Type Conversion2 : DataTypeConversion
  u8ExecutedCycle : Outport
  u8ExcutedStep : Outport  Port=2
  wires:
  Constant1/1 -> Data Type Conversion2/1
  Constant/1 -> Data Type Conversion1/1
  Data Type Conversion1/1 -> u8ExecutedCycle/1
  Data Type Conversion2/1 -> u8ExcutedStep/1

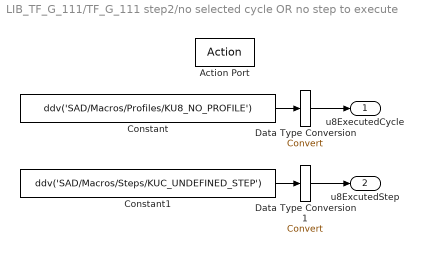
== system LIB_TF_G_111/TF_G_111 step2/no selected cycle OR no step to execute ==
  Action Port : ActionPort
  Constant : Constant  Value=ddv('SAD/Macros/Profiles/KU8_NO_PROFILE')  mask(TL_Constant){data={'output',{'variable','SAD/Macros/Profiles/KU8_NO_PROFILE'},'date',738321.62906249997}}
      settings: CopyFcn=if exist('tl_reset_reviewflag','file')==2,tl_reset_reviewflag(gcbh);end  DeleteFcn=if exist('delete_tlblock','file')==2,delete_tlblock(gcbh);end  NameChangeFcn=if exist('rename_tlblock','file')==2,rename_tlblock(gcbh);end  OpenFcn=if exist('tl_open_blockdlg','file')==2,tl_open_blockdlg(gcbh);else,open_system(gcbh,'parameter');end
      mask Help: eval(['if exist(''tl_online_help'',''file'') == 2, tl_online_help(''Topic'',''TL_Constant''),else, web([''jar:file:///'',matlabroot,''/help/toolbox/simulink/help.jar!/slref/' lower(get_param(gcbh,'Blocktype')) '.html''], ''-helpbrowser''),end'])
      mask Display: plot([-0.05, 1.05, NaN, -0.05, 1.05],[.01, .01, NaN, .99, .99])
  Constant1 : Constant  Value=ddv('SAD/Macros/Steps/KUC_UNDEFINED_STEP')  mask(TL_Constant){data={'output',{'variable','SAD/Macros/Steps/KUC_UNDEFINED_STEP'},'date',738321.62919261574}}
      settings: CopyFcn=if exist('tl_reset_reviewflag','file')==2,tl_reset_reviewflag(gcbh);end  DeleteFcn=if exist('delete_tlblock','file')==2,delete_tlblock(gcbh);end  NameChangeFcn=if exist('rename_tlblock','file')==2,rename_tlblock(gcbh);end  OpenFcn=if exist('tl_open_blockdlg','file')==2,tl_open_blockdlg(gcbh);else,open_system(gcbh,'parameter');end
      mask Help: eval(['if exist(''tl_online_help'',''file'') == 2, tl_online_help(''Topic'',''TL_Constant''),else, web([''jar:file:///'',matlabroot,''/help/toolbox/simulink/help.jar!/slref/' lower(get_param(gcbh,'Blocktype')) '.html''], ''-helpbrowser''),end'])
      mask Display: plot([-0.05, 1.05, NaN, -0.05, 1.05],[.01, .01, NaN, .99, .99])
  Data Type Conversion : DataTypeConversion
  Data Type Conversion1 : DataTypeConversion
  u8ExecutedCycle : Outport
  u8ExcutedStep : Outport  Port=2
  wires:
  Constant/1 -> Data Type Conversion/1
  Constant1/1 -> Data Type Conversion1/1
  Data Type Conversion/1 -> u8ExecutedCycle/1
  Data Type Conversion1/1 -> u8ExcutedStep/1

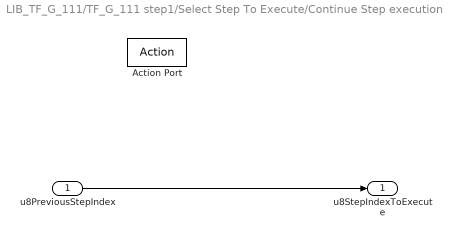
== system LIB_TF_G_111/TF_G_111 step1/Select Step To Execute/Continue Step execution ==
  u8PreviousStepIndex : Inport  RequirementInfo={} %GIDa_fcab27a8_d90a_476c_90c0_241a1e619ec6
  Action Port : ActionPort  RequirementInfo="{}  %GIDa_2c9213f9_d16e_4c91_b642_aee43e9521f1"
  u8StepIndexToExecute : Outport  RequirementInfo={} %GIDa_e09eef44_9847_4a18_ad42_ef98529f821c  InitialOutput=0
  wires:
  u8PreviousStepIndex/1 -> u8StepIndexToExecute/1

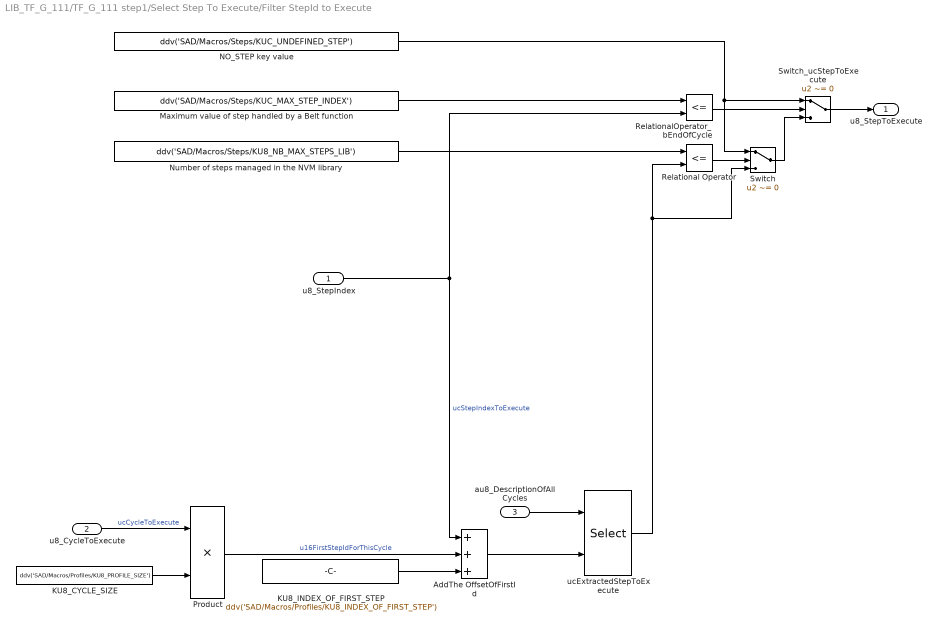
== system LIB_TF_G_111/TF_G_111 step1/Select Step To Execute/Filter StepId to Execute ==
  u8_StepIndex : Inport  RequirementInfo={} %GIDa_7b053a8d_c52f_4f18_a513_21b4e1d02a17  OutDataTypeStr=uint8
  u8_CycleToExecute : Inport  RequirementInfo={} %GIDa_17b8980e_413a_49cb_bbdf_19e5995df7c7  Port=2
  au8_DescriptionOfAllCycles : Inport  RequirementInfo={} %GIDa_914676ae_5bff_4223_821e_99fcbbab0d97  Port=3  OutDataTypeStr=uint8
  AddThe OffsetOfFirstId : Sum  RequirementInfo={} %GIDa_103df495_b24f_4135_8450_3ac2a6ce6256  Inputs=+++  SaturateOnIntegerOverflow=on  OutDataTypeStr=Inherit: Same as first input  mask(TL_Sum){data={'output',{'name','u16StepBytePosition','class','MERGEABLE_GLOBAL','type','UInt16'},'date',738322.64736040507}}
      settings: CopyFcn=if exist('tl_reset_reviewflag','file')==2,tl_reset_reviewflag(gcbh);end  DeleteFcn=if exist('delete_tlblock','file')==2,delete_tlblock(gcbh);end  NameChangeFcn=if exist('rename_tlblock','file')==2,rename_tlblock(gcbh);end  OpenFcn=if exist('tl_open_blockdlg','file')==2,tl_open_blockdlg(gcbh);else,open_system(gcbh,'parameter');end
      mask Help: eval(['if exist(''tl_online_help'',''file'') == 2, tl_online_help(''Topic'',''TL_Sum''),else, web([''jar:file:///'',matlabroot,''/help/toolbox/simulink/help.jar!/slref/' lower(get_param(gcbh,'Blocktype')) '.html''], ''-helpbrowser''),end'])
      mask Display: plot([-0.05, 1.05, NaN, -0.05, 1.05],[.01, .01, NaN, .99, .99])
  KU8_CYCLE_SIZE : Constant  RequirementInfo={} %GIDa_08c4f1ca_bb09_405a_a089_057d29aeb7e1  Value=ddv('SAD/Macros/Profiles/KU8_PROFILE_SIZE')  OutDataTypeStr=Inherit: Inherit via back propagation  mask(TL_Constant){data={'output',{'variable','SAD/Macros/Profiles/KU8_PROFILE_SIZE'},'date',738321.62223840272}}
      settings: CopyFcn=if exist('tl_reset_reviewflag','file')==2,tl_reset_reviewflag(gcbh);end  DeleteFcn=if exist('delete_tlblock','file')==2,delete_tlblock(gcbh);end  NameChangeFcn=if exist('rename_tlblock','file')==2,rename_tlblock(gcbh);end  OpenFcn=if exist('tl_open_blockdlg','file')==2,tl_open_blockdlg(gcbh);else,open_system(gcbh,'parameter');end
      mask Help: eval(['if exist(''tl_online_help'',''file'') == 2, tl_online_help(''Topic'',''TL_Constant''),else, web([''jar:file:///'',matlabroot,''/help/toolbox/simulink/help.jar!/slref/' lower(get_param(gcbh,'Blocktype')) '.html''], ''-helpbrowser''),end'])
      mask Display: plot([-0.05, 1.05, NaN, -0.05, 1.05],[.01, .01, NaN, .99, .99])
  KU8_INDEX_OF_FIRST_STEP : Constant  RequirementInfo={} %GIDa_9066d25c_f8b2_4239_a924_97fad3ec8118  Value=ddv('SAD/Macros/Profiles/KU8_INDEX_OF_FIRST_STEP')  OutDataTypeStr=Inherit: Inherit via back propagation  mask(TL_Constant){data={'output',{'variable','SAD/Macros/Profiles/KU8_INDEX_OF_FIRST_STEP'},'date',738321.62240005785}}
      settings: CopyFcn=if exist('tl_reset_reviewflag','file')==2,tl_reset_reviewflag(gcbh);end  DeleteFcn=if exist('delete_tlblock','file')==2,delete_tlblock(gcbh);end  NameChangeFcn=if exist('rename_tlblock','file')==2,rename_tlblock(gcbh);end  OpenFcn=if exist('tl_open_blockdlg','file')==2,tl_open_blockdlg(gcbh);else,open_system(gcbh,'parameter');end
      mask Help: eval(['if exist(''tl_online_help'',''file'') == 2, tl_online_help(''Topic'',''TL_Constant''),else, web([''jar:file:///'',matlabroot,''/help/toolbox/simulink/help.jar!/slref/' lower(get_param(gcbh,'Blocktype')) '.html''], ''-helpbrowser''),end'])
      mask Display: plot([-0.05, 1.05, NaN, -0.05, 1.05],[.01, .01, NaN, .99, .99])
  Maximum value of step handled by a Belt function : Constant  RequirementInfo={} %GIDa_85e693c4_096a_4e13_a3eb_10d8a1b4db74  Value=ddv('SAD/Macros/Steps/KUC_MAX_STEP_INDEX')  OutDataTypeStr=Inherit: Inherit via back propagation  mask(TL_Constant){data={'output',{'variable','SAD/Macros/Steps/KUC_MAX_STEP_INDEX'},'date',738321.62344370375}}
      settings: CopyFcn=if exist('tl_reset_reviewflag','file')==2,tl_reset_reviewflag(gcbh);end  DeleteFcn=if exist('delete_tlblock','file')==2,delete_tlblock(gcbh);end  NameChangeFcn=if exist('rename_tlblock','file')==2,rename_tlblock(gcbh);end  OpenFcn=if exist('tl_open_blockdlg','file')==2,tl_open_blockdlg(gcbh);else,open_system(gcbh,'parameter');end
      mask Help: eval(['if exist(''tl_online_help'',''file'') == 2, tl_online_help(''Topic'',''TL_Constant''),else, web([''jar:file:///'',matlabroot,''/help/toolbox/simulink/help.jar!/slref/' lower(get_param(gcbh,'Blocktype')) '.html''], ''-helpbrowser''),end'])
      mask Display: plot([-0.05, 1.05, NaN, -0.05, 1.05],[.01, .01, NaN, .99, .99])
  NO_STEP key value : Constant  RequirementInfo={} %GIDa_cb4e9d1a_f250_4569_85fb_c4d5025ec8c8  Value=ddv('SAD/Macros/Steps/KUC_UNDEFINED_STEP')  OutDataTypeStr=uint8  mask(TL_Constant){data={'output',{'variable','SAD/Macros/Steps/KUC_UNDEFINED_STEP'},'date',738321.62358545139}}
      settings: CopyFcn=if exist('tl_reset_reviewflag','file')==2,tl_reset_reviewflag(gcbh);end  DeleteFcn=if exist('delete_tlblock','file')==2,delete_tlblock(gcbh);end  NameChangeFcn=if exist('rename_tlblock','file')==2,rename_tlblock(gcbh);end  OpenFcn=if exist('tl_open_blockdlg','file')==2,tl_open_blockdlg(gcbh);else,open_system(gcbh,'parameter');end
      mask Help: eval(['if exist(''tl_online_help'',''file'') == 2, tl_online_help(''Topic'',''TL_Constant''),else, web([''jar:file:///'',matlabroot,''/help/toolbox/simulink/help.jar!/slref/' lower(get_param(gcbh,'Blocktype')) '.html''], ''-helpbrowser''),end'])
      mask Display: plot([-0.05, 1.05, NaN, -0.05, 1.05],[.01, .01, NaN, .99, .99])
  Number of steps managed in the NVM library : Constant  Value=ddv('SAD/Macros/Steps/KU8_NB_MAX_STEPS_LIB')  mask(TL_Constant){data={'output',{'variable','SAD/Macros/Steps/KU8_NB_MAX_STEPS_LIB'},'date',738321.62256100692}}
      settings: CopyFcn=if exist('tl_reset_reviewflag','file')==2,tl_reset_reviewflag(gcbh);end  DeleteFcn=if exist('delete_tlblock','file')==2,delete_tlblock(gcbh);end  NameChangeFcn=if exist('rename_tlblock','file')==2,rename_tlblock(gcbh);end  OpenFcn=if exist('tl_open_blockdlg','file')==2,tl_open_blockdlg(gcbh);else,open_system(gcbh,'parameter');end
      mask Help: eval(['if exist(''tl_online_help'',''file'') == 2, tl_online_help(''Topic'',''TL_Constant''),else, web([''jar:file:///'',matlabroot,''/help/toolbox/simulink/help.jar!/slref/' lower(get_param(gcbh,'Blocktype')) '.html''], ''-helpbrowser''),end'])
      mask Display: plot([-0.05, 1.05, NaN, -0.05, 1.05],[.01, .01, NaN, .99, .99])
  Product : Product  RequirementInfo={} %GIDa_9d934b81_bf42_4fa9_8243_0cec62096b2c  SaturateOnIntegerOverflow=on  RndMeth=Zero  mask(TL_Product){data={'output',{'type','UInt16'},'date',735951.66832109948}}
      settings: CopyFcn=if exist('tl_reset_reviewflag','file')==2,tl_reset_reviewflag(gcbh);end  DeleteFcn=if exist('delete_tlblock','file')==2,delete_tlblock(gcbh);end  NameChangeFcn=if exist('rename_tlblock','file')==2,rename_tlblock(gcbh);end  OpenFcn=if exist('tl_open_blockdlg','file')==2,tl_open_blockdlg(gcbh);else,open_system(gcbh,'parameter');end
      mask Help: eval(['if exist(''tl_online_help'',''file'') == 2, tl_online_help(''Topic'',''TL_Product''),else, web([''jar:file:///'',matlabroot,''/help/toolbox/simulink/help.jar!/slref/' lower(get_param(gcbh,'Blocktype')) '.html''], ''-helpbrowser''),end'])
      mask Display: plot([-0.05, 1.05, NaN, -0.05, 1.05],[.01, .01, NaN, .99, .99])
  Relational Operator : RelationalOperator  Operator=<=  OutDataTypeStr=boolean  mask(TL_RelationalOperator){data={'date',735951.66832075233}}
      settings: DeleteFcn=if exist('delete_tlblock','file')==2,delete_tlblock(gcbh);end  NameChangeFcn=if exist('rename_tlblock','file')==2,rename_tlblock(gcbh);end  OpenFcn=if exist('tl_open_blockdlg','file')==2,tl_open_blockdlg(gcbh);else,open_system(gcbh,'parameter');end
      mask Help: eval(['if exist(''tl_online_help'',''file'') == 2, tl_online_help(''Topic'',''TL_RelationalOperator''),else, web([''jar:file:///'',matlabroot,''/help/toolbox/simulink/help.jar!/slref/' lower(get_param(gcbh,'Blocktype')) '.html''], ''-helpbrowser''),end'])
      mask Display: plot([-0.05, 1.05, NaN, -0.05, 1.05],[.01, .01, NaN, .99, .99])
  RelationalOperator_bEndOfCycle : RelationalOperator  RequirementInfo={} %GIDa_dee9bedf_e1d6_40ee_a81c_5d5b0d7afec4  Operator=<=  OutDataTypeStr=boolean  mask(TL_RelationalOperator){data={'date',735951.66832049773}}
      settings: DeleteFcn=if exist('delete_tlblock','file')==2,delete_tlblock(gcbh);end  NameChangeFcn=if exist('rename_tlblock','file')==2,rename_tlblock(gcbh);end  OpenFcn=if exist('tl_open_blockdlg','file')==2,tl_open_blockdlg(gcbh);else,open_system(gcbh,'parameter');end
      mask Help: eval(['if exist(''tl_online_help'',''file'') == 2, tl_online_help(''Topic'',''TL_RelationalOperator''),else, web([''jar:file:///'',matlabroot,''/help/toolbox/simulink/help.jar!/slref/' lower(get_param(gcbh,'Blocktype')) '.html''], ''-helpbrowser''),end'])
      mask Display: plot([-0.05, 1.05, NaN, -0.05, 1.05],[.01, .01, NaN, .99, .99])
  Switch : Switch  Criteria=u2 ~= 0  mask(TL_Switch){data={'output',{'type','UInt8'},'date',735951.66832017363}}
      settings: CopyFcn=if exist('tl_reset_reviewflag','file')==2,tl_reset_reviewflag(gcbh);end  DeleteFcn=if exist('delete_tlblock','file')==2,delete_tlblock(gcbh);end  NameChangeFcn=if exist('rename_tlblock','file')==2,rename_tlblock(gcbh);end  OpenFcn=if exist('tl_open_blockdlg','file')==2,tl_open_blockdlg(gcbh);else,open_system(gcbh,'parameter');end
      mask Help: eval(['if exist(''tl_online_help'',''file'') == 2, tl_online_help(''Topic'',''TL_Switch''),else, web([''jar:file:///'',matlabroot,''/help/toolbox/simulink/help.jar!/slref/' lower(get_param(gcbh,'Blocktype')) '.html''], ''-helpbrowser''),end'])
      mask Display: plot([-0.05, 1.05, NaN, -0.05, 1.05],[.01, .01, NaN, .99, .99])
  Switch_ucStepToExecute : Switch  RequirementInfo={} %GIDa_0ccb8e21_1f06_44ba_8891_d931f8a2b0a6  Criteria=u2 ~= 0  mask(TL_Switch){data={'output',{'type','UInt8'},'threshold',{'scalar',1},'date',738342.71397381939}}
      settings: CopyFcn=if exist('tl_reset_reviewflag','file')==2,tl_reset_reviewflag(gcbh);end  DeleteFcn=if exist('delete_tlblock','file')==2,delete_tlblock(gcbh);end  NameChangeFcn=if exist('rename_tlblock','file')==2,rename_tlblock(gcbh);end  OpenFcn=if exist('tl_open_blockdlg','file')==2,tl_open_blockdlg(gcbh);else,open_system(gcbh,'parameter');end
      mask Help: eval(['if exist(''tl_online_help'',''file'') == 2, tl_online_help(''Topic'',''TL_Switch''),else, web([''jar:file:///'',matlabroot,''/help/toolbox/simulink/help.jar!/slref/' lower(get_param(gcbh,'Blocktype')) '.html''], ''-helpbrowser''),end'])
      mask Display: plot([-0.05, 1.05, NaN, -0.05, 1.05],[.01, .01, NaN, .99, .99])
  ucExtractedStepToExecute : Selector  RequirementInfo={} %GIDa_bd695c60_2cc8_4026_b92d_b2da785cce42  IndexMode=Zero-based  IndexOptions=Index vector (port)  Indices=[1:3]  OutputSizes=1
  u8_StepToExecute : Outport  RequirementInfo={} %GIDa_a67a8c94_0338_4ca4_b46d_81643fc60a5b  InitialOutput=255
  wires:
  Product/1 -> AddThe OffsetOfFirstId/2  "u16FirstStepIdForThisCycle"
  KU8_CYCLE_SIZE/1 -> Product/2
  KU8_INDEX_OF_FIRST_STEP/1 -> AddThe OffsetOfFirstId/3
  AddThe OffsetOfFirstId/1 -> ucExtractedStepToExecute/2
  RelationalOperator_bEndOfCycle/1 -> Switch_ucStepToExecute/2
  NO_STEP key value/1 -> Switch_ucStepToExecute/1, Switch/1
  u8_CycleToExecute/1 -> Product/1  "ucCycleToExecute"
  au8_DescriptionOfAllCycles/1 -> ucExtractedStepToExecute/1
  Switch_ucStepToExecute/1 -> u8_StepToExecute/1
  Maximum value of step handled by a Belt function/1 -> RelationalOperator_bEndOfCycle/1
  Switch/1 -> Switch_ucStepToExecute/3
  Relational Operator/1 -> Switch/2
  Number of steps managed in the NVM library/1 -> Relational Operator/1
  ucExtractedStepToExecute/1 -> Switch/3, Relational Operator/2
  u8_StepIndex/1 -> RelationalOperator_bEndOfCycle/2, AddThe OffsetOfFirstId/1  "ucStepIndexToExecute"

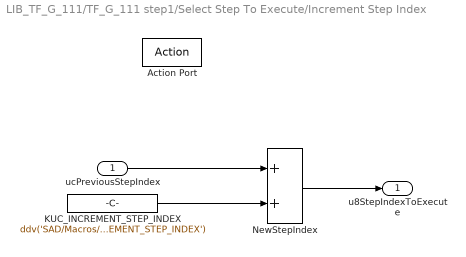
== system LIB_TF_G_111/TF_G_111 step1/Select Step To Execute/Increment Step Index ==
  ucPreviousStepIndex : Inport  RequirementInfo={} %GIDa_4cd58760_9ad1_4752_8fa3_fbb737a7480a
  Action Port : ActionPort  RequirementInfo="{}  %GIDa_54631830_eabe_46a1_add0_fae64ef8c3bc"
  KUC_INCREMENT_STEP_INDEX : Constant  RequirementInfo={} %GIDa_79068a5a_3d13_4a18_b0fc_31166480a7ba  Value=ddv('SAD/Macros/Steps/KUC_INCREMENT_STEP_INDEX')  OutDataTypeStr=Inherit: Inherit via back propagation  mask(TL_Constant){data={'output',{'variable','SAD/Macros/Steps/KUC_INCREMENT_STEP_INDEX'},'date',738321.62125100696}}
      settings: CopyFcn=if exist('tl_reset_reviewflag','file')==2,tl_reset_reviewflag(gcbh);end  DeleteFcn=if exist('delete_tlblock','file')==2,delete_tlblock(gcbh);end  NameChangeFcn=if exist('rename_tlblock','file')==2,rename_tlblock(gcbh);end  OpenFcn=if exist('tl_open_blockdlg','file')==2,tl_open_blockdlg(gcbh);else,open_system(gcbh,'parameter');end
      mask Help: eval(['if exist(''tl_online_help'',''file'') == 2, tl_online_help(''Topic'',''TL_Constant''),else, web([''jar:file:///'',matlabroot,''/help/toolbox/simulink/help.jar!/slref/' lower(get_param(gcbh,'Blocktype')) '.html''], ''-helpbrowser''),end'])
      mask Display: plot([-0.05, 1.05, NaN, -0.05, 1.05],[.01, .01, NaN, .99, .99])
  NewStepIndex : Sum  RequirementInfo={} %GIDa_df793995_a6cc_4c65_9ff1_a03c2377833c  OutDataTypeStr=Inherit: Inherit via back propagation  mask(TL_Sum){data={'output',{'name','u8NewStepIndex','type','UInt8'},'date',735951.66831876163}}
      settings: AttributesFormatString=Saturation: %<SaturateOnIntegerOverflow>  CopyFcn=if exist('tl_reset_reviewflag','file')==2,tl_reset_reviewflag(gcbh);end  DeleteFcn=if exist('delete_tlblock','file')==2,delete_tlblock(gcbh);end  NameChangeFcn=if exist('rename_tlblock','file')==2,rename_tlblock(gcbh);end  OpenFcn=if exist('tl_open_blockdlg','file')==2,tl_open_blockdlg(gcbh);else,open_system(gcbh,'parameter');end
      mask Help: eval(['if exist(''tl_online_help'',''file'') == 2, tl_online_help(''Topic'',''TL_Sum''),else, web([''jar:file:///'',matlabroot,''/help/toolbox/simulink/help.jar!/slref/' lower(get_param(gcbh,'Blocktype')) '.html''], ''-helpbrowser''),end'])
      mask Display: plot([-0.05, 1.05, NaN, -0.05, 1.05],[.01, .01, NaN, .99, .99])
  u8StepIndexToExecute : Outport  RequirementInfo={} %GIDa_6380abbd_d589_46e0_9418_0b26f4160665  InitialOutput=0
  wires:
  KUC_INCREMENT_STEP_INDEX/1 -> NewStepIndex/2
  ucPreviousStepIndex/1 -> NewStepIndex/1
  NewStepIndex/1 -> u8StepIndexToExecute/1

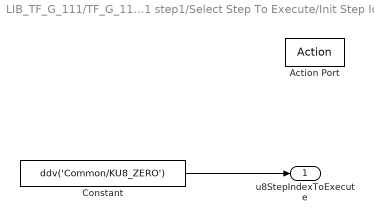
== system LIB_TF_G_111/TF_G_111 step1/Select Step To Execute/Init Step Id ==
  Action Port : ActionPort  RequirementInfo="{}  %GIDa_a1b0021c_7f73_45c2_aadd_b61db888fbe6"
  Constant : Constant  RequirementInfo={} %GIDa_7ece66ff_aed8_4357_a2d7_da4c23e09d80  Value=ddv('Common/KU8_ZERO')  OutDataTypeStr=uint8  mask(TL_Constant){data={'output',{'variable','Common/KU8_ZERO'},'autoscaling',{'mode',2,'scalingvalid',1},'date',735951.66831836803}}
      settings: CopyFcn=if exist('tl_reset_reviewflag','file')==2,tl_reset_reviewflag(gcbh);end  DeleteFcn=if exist('delete_tlblock','file')==2,delete_tlblock(gcbh);end  NameChangeFcn=if exist('rename_tlblock','file')==2,rename_tlblock(gcbh);end  OpenFcn=if exist('tl_open_blockdlg','file')==2,tl_open_blockdlg(gcbh);else,open_system(gcbh,'parameter');end
      mask Help: eval(['if exist(''tl_online_help'',''file'') == 2, tl_online_help(''Topic'',''TL_Constant''),else, web([''jar:file:///'',matlabroot,''/help/toolbox/simulink/help.jar!/slref/' lower(get_param(gcbh,'Blocktype')) '.html''], ''-helpbrowser''),end'])
      mask Display: plot([-0.05, 1.05, NaN, -0.05, 1.05],[.01, .01, NaN, .99, .99])
  u8StepIndexToExecute : Outport  RequirementInfo={} %GIDa_0b043a17_cf3e_4676_838c_da1c1d40acda  OutDataTypeStr=uint8  InitialOutput=0
  wires:
  Constant/1 -> u8StepIndexToExecute/1
